simulink model "PID_Controller"  (Simulink 5.0)
settings: Solver=ode45  StartTime=0.0  StopTime=10  FixedStep=0.1  MaxStep=0.001  RelTol=1e-9  AbsTol=1e-12
values from neighbouring files (symbols this model uses):
  delay = 0.001    [FIGURES.M]
  integ_threshold = 0.1    [FIGURES.M]
  Kd = 0.8    [FIGURES.M]
  Ki = 0.1    [FIGURES.M]
  Kp = 10    [FIGURES.M]
  limit = 0.5    [FIGURES.M]
settings Model: LastModifiedBy=Administrator  BooleanDataType=off

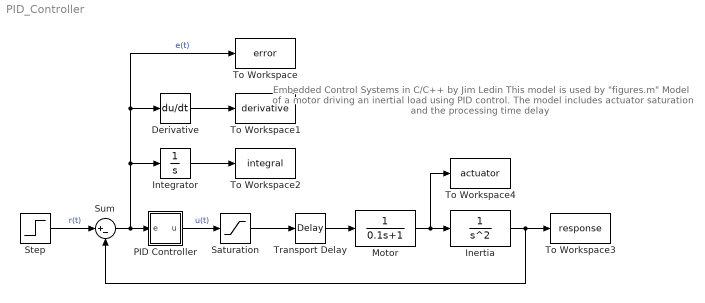
== system PID_Controller ==
  note: Embedded Control Systems in C/C++
      | by Jim Ledin
      |
      | This model is used by "figures.m"
      |
      | Model of a motor driving an inertial load
      | using PID control.
      | The model includes actuator saturation
      | and the processing time delay
  Derivative : Derivative
  Inertia : TransferFcn  Denominator=[1 0 0]
  Integrator : Integrator
  Motor : TransferFcn  Denominator=[0.1 1]
  PID Controller : Subsystem  AncestorBlock=simulink_extras/Additional Linear/PID Controller  mask(PID Controller){Kp=Kp, Ki=Ki, Kd=Kd, windup_limit=integ_threshold}
      mask prompts: Kp "Proportional Gain:"; Ki "Integral Gain:"; Kd "Derivative Gain:"; windup_limit "Windup Error Threshold:"
      mask help:
      | Enter expressions for proportional, integral, and derivative gains and for the integrator windup error threshold.
      | u = Kp(Ki/s + Kds + 1) e
  Saturation : Saturate  UpperLimit=limit  LowerLimit=-limit
  Step : Step  Time=0  SampleTime=0
  Sum : Sum  Inputs=|+-  SaturateOnIntegerOverflow=on  InputSameDT=on
  To Workspace : ToWorkspace  VariableName=error  SampleTime=-1  SaveFormat=StructureWithTime
  To Workspace1 : ToWorkspace  VariableName=derivative  SampleTime=-1  SaveFormat=StructureWithTime
  To Workspace2 : ToWorkspace  VariableName=integral  SampleTime=-1  SaveFormat=StructureWithTime
  To Workspace3 : ToWorkspace  VariableName=response  SampleTime=-1  SaveFormat=StructureWithTime
  To Workspace4 : ToWorkspace  VariableName=actuator  SampleTime=-1  SaveFormat=StructureWithTime
  Transport Delay : TransportDelay  DelayTime=delay
  wires:
  Inertia/1 -> To Workspace3/1, Sum/2
  Sum/1 -> Integrator/1, To Workspace/1, Derivative/1, PID Controller/1(e)  "e(t)"
  Step/1 -> Sum/1  "r(t)"
  Motor/1 -> Inertia/1, To Workspace4/1
  Integrator/1 -> To Workspace2/1
  Derivative/1 -> To Workspace1/1
  PID Controller/1(u) -> Saturation/1  "u(t)"
  Saturation/1 -> Transport Delay/1
  Transport Delay/1 -> Motor/1

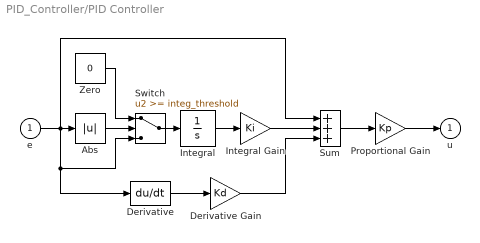
== system PID_Controller/PID Controller ==
  e : Inport
  Abs : Abs  SaturateOnIntegerOverflow=on
  Derivative : Derivative
  Derivative Gain : Gain  Gain=Kd  SaturateOnIntegerOverflow=on
  Integral : TransferFcn  Numerator=1  Denominator=[1 0]
  Integral Gain : Gain  Gain=Ki  SaturateOnIntegerOverflow=on
  Proportional Gain : Gain  Gain=Kp  SaturateOnIntegerOverflow=on
  Sum : Sum  Inputs=+++  SaturateOnIntegerOverflow=on  InputSameDT=on
  Switch : Switch  Threshold=integ_threshold  SaturateOnIntegerOverflow=on  InputSameDT=on
  Zero : Constant  Value=0
  u : Outport  InitialOutput=0
  wires:
  Integral/1 -> Integral Gain/1
  Derivative Gain/1 -> Sum/3
  e/1 -> Sum/1, Derivative/1, Switch/3, Abs/1
  Sum/1 -> Proportional Gain/1
  Derivative/1 -> Derivative Gain/1
  Proportional Gain/1 -> u/1
  Integral Gain/1 -> Sum/2
  Switch/1 -> Integral/1
  Abs/1 -> Switch/2
  Zero/1 -> Switch/1
